simulink model "purepursuit_adv"  (R2025b)
settings: Solver=ode8  StartTime=0.0  StopTime=240  FixedStep=0.05  RelTol=1e-3
values from neighbouring files (symbols this model uses):
  maxNoise = 0.000001    (= 1e-06)    [pathTracking_main.m]
  minNoise = -0.0000001    (= -1e-07)    [pathTracking_main.m]
libraries: matrix_library x2
settings Model: Creator=ockap  LastModifiedBy=Riley Martin
settings OptimizationCC: DefaultParameterBehavior=Inlined  UseDivisionForNetSlopeComputation=on  GainParamInheritBuiltInType=on  UseFloatMulNetSlope=on  InlineInvariantSignals=on  PassReuseOutputArgsAs=Individual arguments  ZeroExternalMemoryAtStartup=off  ZeroInternalMemoryAtStartup=off  NoFixptDivByZeroProtection=on  EfficientFloat2IntCast=on  LifeSpan=1  OptimizeBlockOrder=speed  DifferentSizesBufferReuse=on  EfficientTunableParamExpr=on
settings DebuggingCC: ParameterTunabilityLossMsg=error
settings HardwareCC: ProdLongLongMode=on
settings SFSimCC: MATLABDynamicMemAlloc=off
settings RTWCC: SystemTargetFile=ert.tlc  GenCodeOnly=on  TemplateMakefile=ert_default_tmf  TargetLang=C++  GPUComputeCapability=3.5  Description=Embedded Coder
settings CodeAppCC: ForceParamTrailComments=on  IgnoreCustomStorageClasses=off  OperatorAnnotations=on  SimulinkDataObjDesc=on  SFDataObjDesc=on  CustomSymbolStrGlobalVar=rt$N$M  CustomSymbolStrType=$N$M  CustomSymbolStrFcn=$N$M$F  CustomSymbolStrMacro=$N$M  InsertBlockDesc=on
settings ERTTargetCC: RootIOFormat=Structure reference  ERTCustomFileTemplate=example_file_process.tlc  ERTFilePackagingFormat=CompactWithDataFile  TargetLangStandard=C++11 (ISO)  GenerateSampleERTMain=on  IncludeMdlTerminateFcn=off  CombineSignalStateStructs=on  SupportAbsoluteTime=off  CodeInterfacePackaging=C++ class  SubcomponentCodeInterfacePackaging=C++ class  SupportComplex=off  SupportContinuousTime=on  SupportNonInlinedSFcns=on

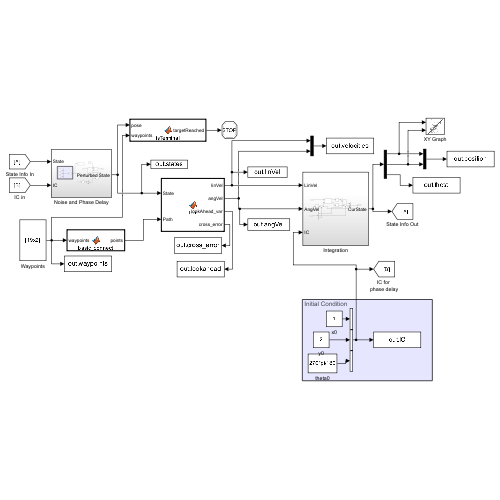
[thumbnail: Simulink's stored preview of the top-level diagram]
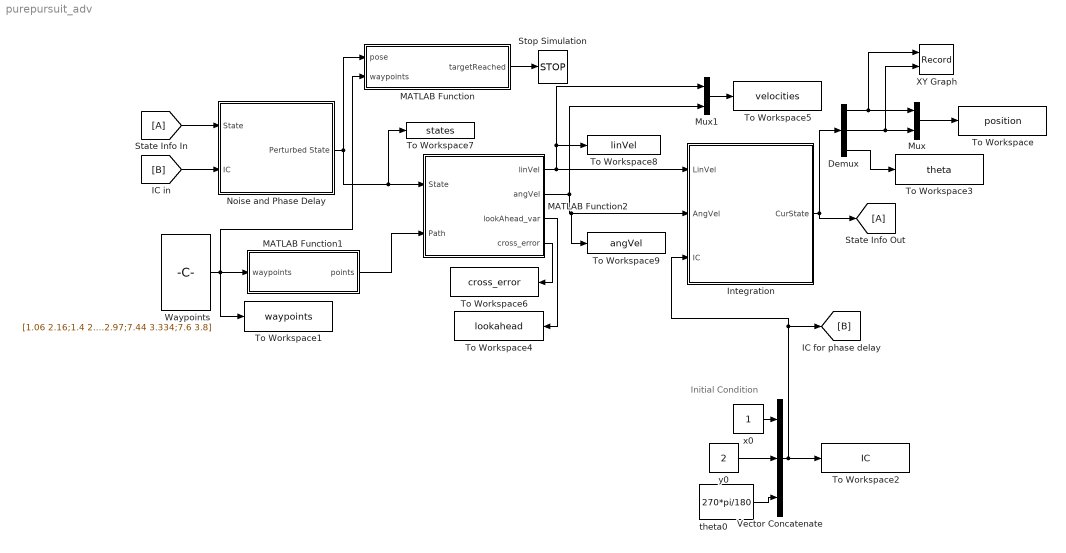
== system purepursuit_adv ==
  note: Initial Condition
  Demux : Demux  Outputs=3
  Integration : Subsystem
  MATLAB Function : MATLAB Function  TreatAsAtomicUnit=on
  MATLAB Function1 : MATLAB Function  TreatAsAtomicUnit=on
  MATLAB Function2 : MATLAB Function  TreatAsAtomicUnit=on  SystemSampleTime=0.1
  Mux : Mux  Inputs=2
  Mux1 : Mux  Inputs=2
  Noise and Phase Delay : Subsystem
  State Info In : From
  State Info Out : Goto
  Stop Simulation : Stop
  To Workspace : ToWorkspace  VariableName=position  SaveFormat=Timeseries  SampleTime=-1
  To Workspace1 : ToWorkspace  VariableName=waypoints  SaveFormat=Structure With Time  SampleTime=-1
  To Workspace2 : ToWorkspace  VariableName=IC  SampleTime=-1
      settings: Save2DSignal=2-D array (concatenate along first dimension)
  To Workspace3 : ToWorkspace  VariableName=theta  SaveFormat=Timeseries  SampleTime=-1
  To Workspace4 : ToWorkspace  VariableName=lookahead  SaveFormat=Structure  SampleTime=-1
  To Workspace5 : ToWorkspace  VariableName=velocities  SaveFormat=Structure With Time  SampleTime=-1
  To Workspace6 : ToWorkspace  VariableName=cross_error  SaveFormat=Structure  SampleTime=-1
  To Workspace7 : ToWorkspace  VariableName=states  SaveFormat=Structure With Time  SampleTime=-1
  To Workspace8 : ToWorkspace  VariableName=linVel  SaveFormat=Structure With Time  SampleTime=-1
  To Workspace9 : ToWorkspace  VariableName=angVel  SaveFormat=Structure With Time  SampleTime=-1
  Vector Concatenate : Concatenate  NumInputs=3
  Waypoints : Constant  Value=[1.06 2.16;1.4 2.4;1.72 2.744;1.966 3.06;2.336 3.363;2.73 3.45;3.185 3.25;3.74 3.22;4.02 3.64;4.39 4.12;5.02 4.25;5.556 3.96;5.86 3.6;6 3.2;6.37 2.75;6.96 2.58;7.32 2.97;7.44 3.334;7.6 3.8]  VectorParams1D=off  SampleTime=-1
  XY Graph : Record  NumPorts=2.0  FileSettingsInternal="{\"entries\":[{\"content\":{\"excelSettings\":{\"content\":{},\"type\":\"Streamout.ExcelSettings\"},\"parquetSettings\":{\"content\":{},\"type\":\"Streamout.ParquetSettings\"}},\"type\":\"Streamout.FileSettingStorage\",\"uuid\":\"\"}],\"packageUris\":[\"http:\\/\\/schema.mathworks.com\\/mf0\\/streamout_blocks\\/R2020a\"],\"version\":\"1.0\"}"  FrameSettings=[0, 0]  Layout=[1 1]  SignalsInternal="{\"entries\":[{\"content\":{\"signals\":[{\"content\":{\"blockPath\":[],\"dimensions\":[1],\"domain\":\"\",\"lineColor\":\"#a2142f\",\"plots\":[ 1 ],\"port\":1,\"sid\":[\"\"],\"signalID\":1,\"signalName\":\"Demux:1\"},\"type\":\"RecordBlkView.Signal\",\"uuid\":\"\"},{\"content\":{\"blockPath\":[],\"dimensions\":[1],\"domain\":\"\",\"lineColor\":\"#139fff\",\"plots\":[ 1 ],\"port\":2,\"sid\":[\"\"],\"signalID\":2,\"signalName\":\"Demux:2\"},\"type\":\"RecordBlkView.Signal\",\"uuid\":\"\"}]},\"type\":\"RecordBlkView.InputSignals\",\"uuid\":\"\"}],\"packageUris\":[\"http:\\/\\/schema.mathworks.com\\/mf0\\/streamout_blocks\\/R2020a\"],\"version\":\"1.0\"}"  VisualizationBindings="{\"xyplotplugin\":{\"info\":[{\"series\":[{\"bindingParametersList\":[{\"parameter\":\"X-Axis\",\"signalID\":1,\"signalName\":\"Demux:1\"},{\"parameter\":\"Y-Axis\",\"signalID\":2,\"signalName\":\"Demux:2\"}],\"seriesID\":0}],\"subplotID\":1}]}}"  CompatibilityTag=XY
  theta0 : Constant  Value=270*pi/180
  x0 : Constant
  y0 : Constant  Value=2
  wires:
  Demux/1 -> XY Graph/1, Mux/1
  Demux/2 -> XY Graph/2, Mux/2
  Demux/3 -> To Workspace3/1
  Mux/1 -> To Workspace/1
  Vector Concatenate/1 -> To Workspace2/1, Integration/3(IC), [B]
  x0/1 -> Vector Concatenate/1
  Integration/1(CurState) -> Demux/1, State Info Out/1
  y0/1 -> Vector Concatenate/2
  [B] -> Noise and Phase Delay/2(IC)
  theta0/1 -> Vector Concatenate/3
  State Info In/1 -> Noise and Phase Delay/1(State)
  Noise and Phase Delay/1(Perturbed State) -> MATLAB Function/1(pose), To Workspace7/1, MATLAB Function2/1(State)
  MATLAB Function/1(targetReached) -> Stop Simulation/1
  Waypoints/1 -> To Workspace1/1, MATLAB Function1/1(waypoints), MATLAB Function/2(waypoints)
  MATLAB Function1/1(points) -> MATLAB Function2/2(Path)
  MATLAB Function2/3(lookAhead_var) -> To Workspace4/1
  Mux1/1 -> To Workspace5/1
  MATLAB Function2/1(linVel) -> To Workspace8/1, Mux1/1, Integration/1(LinVel)
  MATLAB Function2/4(cross_error) -> To Workspace6/1
  MATLAB Function2/2(angVel) -> Mux1/2, Integration/2(AngVel), To Workspace9/1

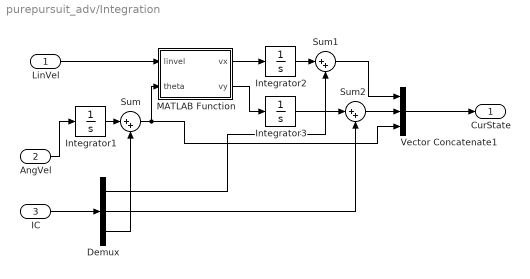
== system purepursuit_adv/Integration ==
  LinVel : Inport
  AngVel : Inport  Port=2
  IC : Inport  Port=3
  Demux : Demux  Outputs=3
  Integrator1 : Integrator
  Integrator2 : Integrator
  Integrator3 : Integrator
  MATLAB Function : MATLAB Function  TreatAsAtomicUnit=on
  Sum : Sum  Inputs=|++
  Sum1 : Sum  Inputs=|++
  Sum2 : Sum  Inputs=|++
  Vector Concatenate1 : Concatenate  NumInputs=3
  CurState : Outport
  wires:
  MATLAB Function/1(vx) -> Integrator2/1
  MATLAB Function/2(vy) -> Integrator3/1
  AngVel/1 -> Integrator1/1
  LinVel/1 -> MATLAB Function/1(linvel)
  Vector Concatenate1/1 -> CurState/1
  Integrator1/1 -> Sum/1
  Demux/3 -> Sum/2
  Integrator2/1 -> Sum1/1
  Demux/1 -> Sum1/2
  Demux/2 -> Sum2/2
  Integrator3/1 -> Sum2/1
  Sum2/1 -> Vector Concatenate1/2
  Sum1/1 -> Vector Concatenate1/1
  IC/1 -> Demux/1
  Sum/1 -> MATLAB Function/2(theta), Vector Concatenate1/3

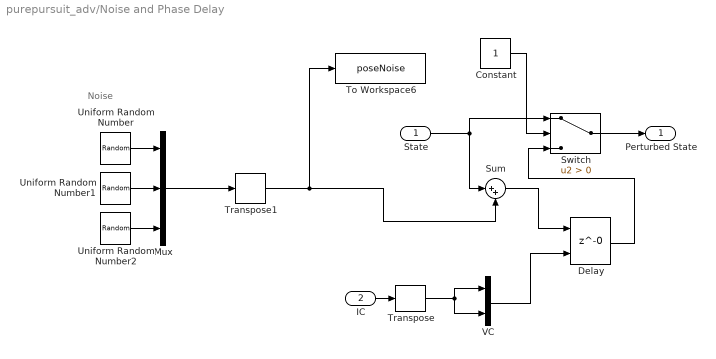
== system purepursuit_adv/Noise and Phase Delay ==
  note: Noise
  State : Inport
  IC : Inport  Port=2
  Constant : Constant
  Delay : Delay  DelayLength=0  InitialConditionSource=Input port  InitialCondition=0  InputProcessing=Columns as channels (frame based)
      settings: InputPortMap=u0,p4
  Mux : Mux  Inputs=3
  Sum : Sum  Inputs=|++
  Switch : Switch  Criteria=u2 > Threshold  SaturateOnIntegerOverflow=off  InputSameDT=off
  To Workspace6 : ToWorkspace  VariableName=poseNoise  SampleTime=-1
      settings: Save2DSignal=2-D array (concatenate along first dimension)
  Transpose : matrix_library/Transpose
  Transpose1 : matrix_library/Transpose
  Uniform Random Number : UniformRandomNumber  Minimum=minNoise  Maximum=maxNoise  SampleTime=0.1
  Uniform Random Number1 : UniformRandomNumber  Minimum=minNoise  Maximum=maxNoise  SampleTime=0.1
  Uniform Random Number2 : UniformRandomNumber  Minimum=minNoise  Maximum=maxNoise  SampleTime=0.1
  VC : Concatenate  Mode=Multidimensional array
  Perturbed State : Outport
  wires:
  IC/1 -> Transpose/1
  Transpose1/1 -> Sum/2, To Workspace6/1
  Transpose/1 -> VC/2, VC/1
  VC/1 -> Delay/2
  Uniform Random Number2/1 -> Mux/3
  Uniform Random Number1/1 -> Mux/2
  Uniform Random Number/1 -> Mux/1
  Mux/1 -> Transpose1/1
  Sum/1 -> Delay/1
  State/1 -> Switch/1, Sum/1
  Switch/1 -> Perturbed State/1
  Delay/1 -> Switch/3
  Constant/1 -> Switch/2

== matlab function purepursuit_adv/MATLAB Function ==
  data: pose input; targetReached output; waypoints input
function targetReached = isTerminal(pose,waypoints)
    distance = norm(pose(1:2) - waypoints(end,:));
    targetReached = 0;
    if(distance < 0.03)
        targetReached = 1;
    end

== matlab function purepursuit_adv/Integration/MATLAB Function ==
  data: linvel input; vx output; theta input; vy output
function [vx,vy] = fcn(linvel,theta)
    vx = linvel*cos(theta);
    vy = linvel*sin(theta);
end

== matlab function purepursuit_adv/MATLAB Function1 ==
  data: waypoints input; points output
function points = basic_connect(waypoints)
    
    % parameter t
    t = 1:length(waypoints(:,1));
    
    % create parametric splines
    tq = linspace(1,length(waypoints(:,1)),200);  % many samples for smooth curve
    xs = spline(t, waypoints(:,1), tq);
    ys = spline(t, waypoints(:,2), tq);

    points = zeros(length(xs),2);

    points(:,1) = xs;
    points(:,2) = ys;

end

% function points = basic_connect(waypoints)
% %#codegen
% % Works in Simulink with fixed-size signals (no variable-size settings)
% 
% MAX_POINTS = 400;     % total number of points in output
% RESOLUTION = 0.1;     % interpolation step (units)
% POINTS_PER_SEGMENT = 50; % fixed number of points per segment (avoid variable length)
% 
% points = zeros(MAX_POINTS, 2);  % fixed-size output
% counter = 1;
% 
% for i = 2:size(waypoints,1)
%     % Compute differences
%     delta_x = waypoints(i,1) - waypoints(i-1,1);
%     delta_y = waypoints(i,2) - waypoints(i-1,2);
% 
%     % Use a fixed number of interpolation points per segment
%     num_points = POINTS_PER_SEGMENT;
% 
%     % Generate evenly spaced points (fixed length)
%     x_points = linspace(waypoints(i-1,1), waypoints(i,1), num_points);
%     y_points = linspace(waypoints(i-1,2), waypoints(i,2), num_points);
% 
%     % Determine where to store them in the fixed output matrix
%     end_idx = min(counter + num_points - 1, MAX_POINTS);
% 
%     % Copy into output (truncate if necessary)
%     valid_length = end_idx - counter + 1;
%     points(counter:end_idx, 1) = x_points(1:valid_length);
%     points(counter:end_idx, 2) = y_points(1:valid_length);
% 
%     counter = end_idx + 1;
%     if counter > MAX_POINTS
%         break; % stop if buffer is full
%     end
% end
% end

== matlab function purepursuit_adv/MATLAB Function2 ==
  data: State input; Path input; linVel output; angVel output; lookAhead_var output; cross_error output
function [linVel, angVel, lookAhead_var, cross_error] = fcn(State, Path)
% State = [x, y, yaw]
% Path = [x_path, y_path]
% lookAhead = lookahead distance (m)
% linVel = forward speed (m/s)
    
    % DECLARE PERSISTENT VARIABLE to hold the last closest index
    % Initialize it to 1 the first time the function runs
    persistent last_refindex;
    if isempty(last_refindex)
        last_refindex = 1;
    end
    
    % Break Path into x and y
    x = Path(:,1);
    y = Path(:,2);
    
    % Derivatives for curvature (Unchanged)
    dx = gradient(x);
    dy = gradient(y);
    ddx = gradient(dx);
    ddy = gradient(dy);
    
    % Path curvature
    K = (dx .* ddy - dy .* ddx) ./ ((dx.^2 + dy.^2).^(3/2));
    
    % Variable lookahead (Unchanged)
    K_norm = (K - min(K)) / (max(K) - min(K));
    invK = 1 - K_norm;
    L_min = 0.05;
    L_max = 0.15;
    
    lookAhead_var = L_min + invK * (L_max - L_min);

    % Variable lookahead (Unchanged)
    linV_min = 0.05;
    linV_max = 0.2;
    
    %linVel_vec = 0.15;
    linVel_vec = linV_min + invK * (linV_max - linV_min);

    % Rear axle midpoint
    backWheel_pos = [State(1) + cos(State(3))*0.15, ...
                     State(2) + sin(State(3))*0.15];
    
    % Distance from all path points to rear axle
    delta_x = Path(:,1) - backWheel_pos(1);
    delta_y = Path(:,2) - backWheel_pos(2);
    dists = sqrt(delta_x.^2 + delta_y.^2);

    % --- FIX: Restrict the search space to maintain forward progress ---
    
    % 1. Create a subset of the path starting from the last known closest point.
    % We only want to search path points from `last_refindex` onwards.
    search_dists = dists(last_refindex:end);
    
    % 2. Find the index of the closest point within this restricted subset.
    [~, relative_refindex] = min(search_dists);
    
    % 3. Convert the relative index back to the absolute index for the whole Path array.
    refindex = (last_refindex - 1) + relative_refindex;
    
    % 4. Update the persistent variable for the next time step.
    last_refindex = refindex;

    % --- Find goal point ahead of vehicle (Adjusted to use the new refindex) ---
    
    % validIdx is the first point that is >= lookahead distance AND
    % is at or after the closest point (refindex).

    validIdx = find((dists >= lookAhead_var(refindex)) & (1:length(Path))' >= refindex, 1, 'first');
    
    % Safeguards
    if isempty(validIdx)
        % If no point is far enough, use the last path point as the goal
        validIdx = length(Path);
    end
    
    % Goal position
    goal = Path(validIdx, :);
    
    % Steering angle computation (Unchanged)
    linVel = linVel_vec(refindex); % scalar for this timestep
    alpha = atan2(goal(2) - backWheel_pos(2), goal(1) - backWheel_pos(1)) - State(3);
    alpha = atan2(sin(alpha), cos(alpha));  % normalize between -pi, pi
    kappa = 2 * sin(alpha) / lookAhead_var(refindex);
    
    % Angular velocity
    angVel = linVel .* kappa;

    wpdistances = Path - [State(1)*ones(height(Path),1) State(2)*ones(height(Path),1)];
    [cross_error,refindex] = min(vecnorm(wpdistances,2,2));
end
